simulink model "PF_blok"  (R2023a)
settings: Solver=VariableStepAuto  StartTime=0.0  StopTime=10.0  RelTol=1e-3
settings Model: Creator=user  LastModifiedBy=user

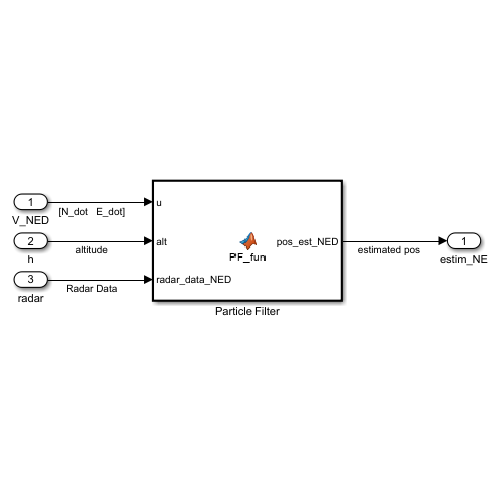
[thumbnail: Simulink's stored preview of the top-level diagram]
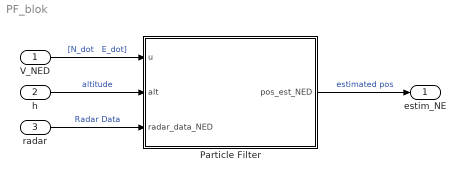
== system PF_blok ==
  V_NED : Inport
  h : Inport  Port=2
  radar : Inport  Port=3
  Particle Filter : MATLAB Function  TreatAsAtomicUnit=on
  estim_NE : Outport
  wires:
  V_NED/1 -> Particle Filter/1(u)  "[N_dot   E_dot]"
  radar/1 -> Particle Filter/3(radar_data_NED)  "Radar Data"
  h/1 -> Particle Filter/2(alt)  "altitude"
  Particle Filter/1(pos_est_NED) -> estim_NE/1  "estimated pos"

== matlab function PF_blok/Particle Filter ==
  data: u input; alt input; pos_est_NED output; radar_data_NED input
function pos_est_NED  = PF_fun(u, alt, radar_data_NED)

% input vector consist of V_N and V_E, those 2 array will be used for
% particles movement through particles kinematic model
% u = [V_N  V_E]; % input vector

% pos_cur_NED = current position of aircraft in NED

% Radar Data
% Radar Data is a 3D array that size is 81x3xSimArray. Unity radar model is
% raycasting throught DTED model with 9x9 square radar beam. Radar Data
% store each 81 points NED position relative to aircraft that touch to DTED surface.
% Those Radar Data will be used for measuring particles DTED altitude when
% they spread in sampling space through interpolation from DTED model.
% radar_data_NED = 81x3

% Move particles for Particle Filter algorithm with u matrix 
PF.particle_step(u);

% Update weights of Particles based on real data value
PF.update_weights(radar_data_NED, alt, dted_grid)

% Take mean and var variable for estimation metrics
[pos_est_NED, var] = PF.estimate();

end
